simulink model "Quadrocopter_control"  (Simulink 7.4)
settings: Solver=ode45  StartTime=0.0  StopTime=10.0  RelTol=1e-3
values from neighbouring files (symbols this model uses):
  f1 = (I_y-I_z)/I_x    [quadrocopter_param.m]
  f2 = rot.J_z/I_x    [quadrocopter_param.m]
  f3 = (I_z-I_x)/I_y    [quadrocopter_param.m]
  f4 = rot.J_z/I_y    [quadrocopter_param.m]
  f5 = (I_x-I_y)/I_z    [quadrocopter_param.m]
  g = 9.81    [quadrocopter_param.m]
  I_x = elec.I_x+bat.I_x+2*boom.I_1x+2*boom.I_1y+2*mot.I_1x+2*mot.I_1y+                             2*rot.I_1x+2*rot.I_1y    [quadrocopter_param.m]
  I_y = elec.I_y+bat.I_y+2*boom.I_1x+2*boom.I_1y+2*mot.I_1x+2*mot.I_1y+                             2*rot.I_1x+2*rot.I_1y    [quadrocopter_param.m]
  I_z = elec.I_z+bat.I_z+4*boom.I_1z+4*mot.I_1z+4*rot.I_1z    [quadrocopter_param.m]
  m = m*1.2    [quadrocopter_param.m]
  phi0 = 0.15    [Quadrocopter_control_Driver.m]    (also in calc_stability.m = 0; control_two_angles_Driver.m; control_two_angles_and_yawrate_Driver.m; discrete_control_phi_theta_rpsi_Driver.m)
  r_phi0 = 0    [Quadrocopter_control_Driver.m]    (also in calc_stability.m; control_two_angles_Driver.m; control_two_angles_and_yawrate_Driver.m; discrete_control_phi_theta_rpsi_Driver.m)
  r_psi0 = 0    [Quadrocopter_control_Driver.m]    (also in calc_stability.m; control_two_angles_Driver.m = 0.01; control_two_angles_and_yawrate_Driver.m = 0.01; discrete_control_phi_theta_rpsi_Driver.m = 0.01)
  r_theta0 = 0    [Quadrocopter_control_Driver.m]    (also in calc_stability.m; control_two_angles_Driver.m; control_two_angles_and_yawrate_Driver.m; discrete_control_phi_theta_rpsi_Driver.m)
  theta0 = 0.15    [Quadrocopter_control_Driver.m]    (also in calc_stability.m = 0; control_two_angles_Driver.m; control_two_angles_and_yawrate_Driver.m; discrete_control_phi_theta_rpsi_Driver.m)
  Ts = 0.005    [quadrocopter_param.m]
undefined symbols (not defined in the file or in its folder): boom, DiscIntNeverNeededParam
libraries: Copter_Library x4, Control_lib x2, simulink x1
settings Model: Creator=roczit00  LastModifiedBy=roczit00

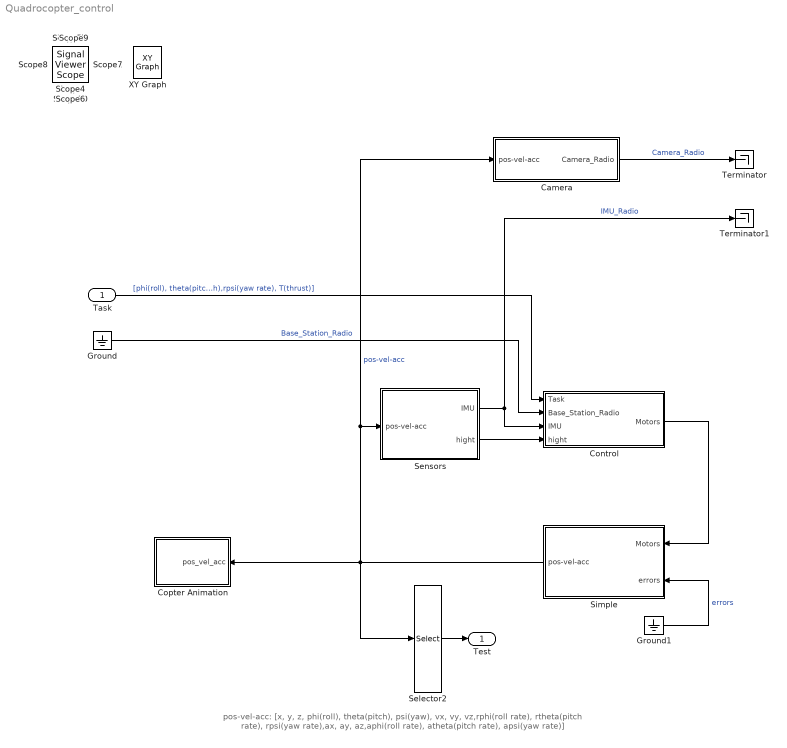
== system Quadrocopter_control ==
  note: pos-vel-acc: [x, y, z, phi(roll), theta(pitch), psi(yaw), vx, vy, vz,rphi(roll rate), rtheta(pitch rate), rpsi(yaw rate),ax, ay, az,aphi(roll rate), atheta(pitch rate), apsi(yaw rate)]
  Task : Inport  PortDimensions=4  OutDataType=fixdt(1, 16)  OutScaling=2^0
  Camera : Subsystem
  Control : Subsystem
  Copter Animation : Subsystem  mask(Quadrocopter Animation){AXES=[-100 100 -100 100 0 100], T_INT=1/25, K_VAR=Feste Position, K_POS=[5 0 1], K_ANGLE=27, A_ON=on, u_phi=on, u_theta=on, u_psi=on, u_x=off, u_y=off, u_z=off}
      mask prompts: AXES "Achsen Grenzen [xmin xmax ymin ymax zmin zmax]"; T_INT "Zeitintervall zwischen Aktualisierungen [s]:"; K_VAR "Kamera Art:"; K_POS "Ort der Kamera [xc yc zc]:"; K_ANGLE "Öffnungswinkel der Kamera [Grad]:"; A_ON "Animation Einschalten:"; u_phi "Use Input phi:"; u_theta "Use Input theta:"; u_psi "Use Input psi:"; u_x "Use Input x:"; u_y "Use Input y:"; u_z "Use Input z:"
      mask help: Erstellt eine 3-D animierte Ansicht eines Quadrocopters.
      mask init:
      | Config.axes = AXES;
      | Config.update = T_INT;
      | Config.camera_view = K_VAR;
      | Config.camera_pos = K_POS;
      | Config.view = K_ANGLE;
      | Config.Animenable = A_ON;
      | Config.phi = u_phi;
      | Config.theta = u_theta;
      | Config.psi = u_psi;
      | Config.x = u_x;
      | Config.y = u_y;
      | Config.z = u_z;
      mask Help:
      | <p>Dieser Block erstellt ein 3 dimensionales Fenster eines Quadrocopters.
      | 
      | <p><H4>Block Eingänge</H4>
      | Der Eingangsvektor bestehend aus:
      | <ul>
      | <li>X-Koordinate - Ort bezogen auf die X-Achse
      | <li>Y-Koordinate - Ort bezogen auf die Y-Achse
      | <li>Z-Koordinate - Ort bezogen auf die Z-Achse
      | <li>Psi - Yaw Drehung um die Z-Achse
      | <li>Phi - Roll Drehen um die Achse in Flugrichtung
      | <li>theta - pitch Neigung in Flugrichtung nach oben bzw. unten
      | </ul></p>
      mask StyleString: edit,edit,popup(Feste Position|Frei bewegbar),edit,edit,checkbox,checkbox,checkbox,checkbox,checkbox,checkbox,checkbox
  Ground : Ground
  Ground1 : Ground
  Selector2 : Selector  InputPortWidth=18  IndexOptions=Index vector (dialog)  Indices=[3 4 5 6]  OutputSizes=1
  Sensors : Subsystem
  Simple : Subsystem  AncestorBlock=Control_lib/Simple
  Terminator : Terminator
  Terminator1 : Terminator
  Test : Outport  OutDataType=fixdt(1, 16)  OutScaling=2^0
  Scope : SignalViewerScope  IOType=viewer  ZoomMode=yonly  LegendLocations="960.3333           681           100      67.33333"  RefreshTime=0.035000
      settings: ShowLegends=on
  Scope1 : SignalViewerScope  IOType=viewer  ZoomMode=yonly  LegendLocations="1037.3333            687             82      67.333333"  RefreshTime=0.035000
      settings: ShowLegends=on
  Scope10 : SignalViewerScope  IOType=viewer  ZoomMode=yonly  LegendLocations="549.3333      405.3333           118            46"  RefreshTime=0.035000
      settings: ShowLegends=on  SaveName=ScopeData10
  Scope2 : SignalViewerScope  IOType=viewer  ZoomMode=yonly  RefreshTime=0.035000
      settings: ShowLegends=on  SaveName=ScopeData2
  Scope3 : SignalViewerScope  IOType=viewer  LegendLocations="235.3333           136            72      67.33333"  RefreshTime=0.035000
      settings: ShowLegends=on  SaveName=ScopeData3
  Scope4 : SignalViewerScope  IOType=viewer  RefreshTime=0.035000
      settings: ShowLegends=on  SaveName=ScopeData4
  Scope5 : SignalViewerScope  IOType=viewer  LegendLocations="401.3333      415.6667           173      192.6667"  RefreshTime=0.035000
      settings: ShowLegends=on  SaveName=ScopeData5
  Scope6 : SignalViewerScope  IOType=viewer  RefreshTime=0.035000
      settings: ShowLegends=on  SaveName=ScopeData6
  Scope7 : SignalViewerScope  IOType=viewer  ZoomMode=yonly  RefreshTime=0.035000
      settings: SaveName=ScopeData7
  Scope8 : SignalViewerScope  IOType=viewer  ZoomMode=yonly  LegendLocations="553.3333      502.3333            92            41"  RefreshTime=0.035000
      settings: ShowLegends=on  SaveName=ScopeData8
  Scope9 : SignalViewerScope  IOType=viewer  LegendLocations="167.3333      162.3333           127            41"  RefreshTime=0.035000
      settings: ShowLegends=on  SaveName=ScopeData9
  XY Graph : simulink/Sinks/XY Graph  IOType=viewer  SystemSampleTime=-1  xmin=-1  xmax=1  ymin=-1  ymax=1  st=-1
  wires:
  Sensors/1(IMU) -> Control/3(IMU), Terminator1/1  "IMU_Radio"
  Sensors/2(hight) -> Control/4(hight)
  Ground1/1 -> Simple/2(errors)  "errors"
  Control/1(Motors) -> Simple/1(Motors)
  Simple/1(pos-vel-acc) -> Sensors/1(pos-vel-acc), Camera/1(pos-vel-acc), Selector2/1, Copter Animation/1(pos_vel_acc)  "pos-vel-acc"
  Camera/1(Camera_Radio) -> Terminator/1  "Camera_Radio"
  Ground/1 -> Control/2(Base_Station_Radio)  "Base_Station_Radio"
  Task/1 -> Control/1(Task)  "[phi(roll), theta(pitch),rpsi(yaw rate), T(thrust)]"
  Selector2/1 -> Test/1

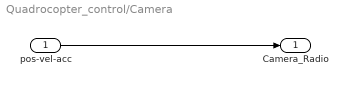
== system Quadrocopter_control/Camera ==
  pos-vel-acc : Inport  OutDataType=fixdt(1, 16)  OutScaling=2^0
  Camera_Radio : Outport  OutDataType=fixdt(1, 16)  OutScaling=2^0
  wires:
  pos-vel-acc/1 -> Camera_Radio/1

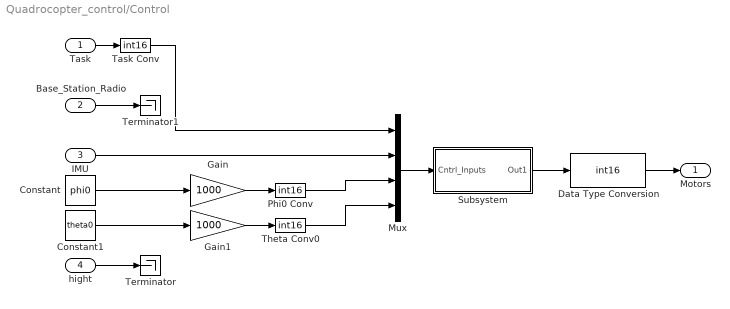
== system Quadrocopter_control/Control ==
  Task : Inport  PortDimensions=4  DataType=double  OutDataType=fixdt(1, 16)  OutScaling=2^0  OutDataTypeStr=double
  Base_Station_Radio : Inport  Port=2  OutDataType=fixdt(1, 16)  OutScaling=2^0
  IMU : Inport  Port=3  DataType=int16  OutDataType=fixdt(1, 16)  OutScaling=2^0  OutDataTypeStr=int16
  hight : Inport  Port=4  DataType=int16  OutDataType=fixdt(1, 16)  OutScaling=2^0  OutDataTypeStr=int16
  Constant : Constant  Value=phi0  OutDataType=fixdt(1, 16)  OutScaling=2^0
  Constant1 : Constant  Value=theta0  OutDataType=fixdt(1, 16)  OutScaling=2^0
  Data Type Conversion : DataTypeConversion  OutDataTypeMode=int16  OutDataType=fixdt(1, 16)  OutScaling=2^0  OutDataTypeStr=int16
  Gain : Gain  Gain=1000  ParameterDataType=fixdt(1, 16)  ParameterScaling=2^0  OutDataType=fixdt(1, 16)  OutScaling=2^0
  Gain1 : Gain  Gain=1000  ParameterDataType=fixdt(1, 16)  ParameterScaling=2^0  OutDataType=fixdt(1, 16)  OutScaling=2^0
  Mux : Mux
  Phi0 Conv : DataTypeConversion  OutDataTypeMode=int16  OutDataType=fixdt(1, 16)  OutScaling=2^0  OutDataTypeStr=int16
  Subsystem : Subsystem  AncestorBlock=Control_lib/Subsystem  mask{G=9.81}
      mask prompts: G "Erdbeschleunigung [m/s²]:"
      mask init:
      | g = G;
  Task Conv : DataTypeConversion  OutDataTypeMode=int16  OutDataType=fixdt(1, 16)  OutScaling=2^0  OutDataTypeStr=int16
  Terminator : Terminator
  Terminator1 : Terminator
  Theta Conv0 : DataTypeConversion  OutDataTypeMode=int16  OutDataType=fixdt(1, 16)  OutScaling=2^0  OutDataTypeStr=int16
  Motors : Outport  PortDimensions=4  DataType=int16  OutDataType=fixdt(1, 16)  OutScaling=2^0  OutDataTypeStr=int16
  wires:
  Base_Station_Radio/1 -> Terminator1/1
  hight/1 -> Terminator/1
  IMU/1 -> Mux/2
  Mux/1 -> Subsystem/1(Cntrl_Inputs)
  Data Type Conversion/1 -> Motors/1
  Subsystem/1(Out1) -> Data Type Conversion/1
  Task/1 -> Task Conv/1
  Task Conv/1 -> Mux/1
  Constant/1 -> Gain/1
  Constant1/1 -> Gain1/1
  Gain/1 -> Phi0 Conv/1
  Gain1/1 -> Theta Conv0/1
  Phi0 Conv/1 -> Mux/3
  Theta Conv0/1 -> Mux/4

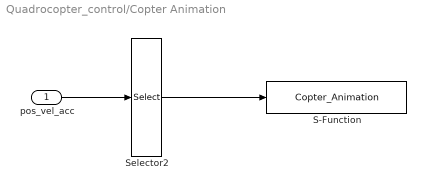
== system Quadrocopter_control/Copter Animation ==
  pos_vel_acc : Inport  PortDimensions=18  OutDataType=sfix(16)  OutScaling=2^0
  S-Function : S-Function  FunctionName=Copter_Animation  Parameters=Config  EnableBusSupport=off
  Selector2 : Selector  InputPortWidth=18  IndexOptions=Index vector (dialog)  Indices=[1 2 3 4 5 6]  OutputSizes=1
  wires:
  pos_vel_acc/1 -> Selector2/1
  Selector2/1 -> S-Function/1

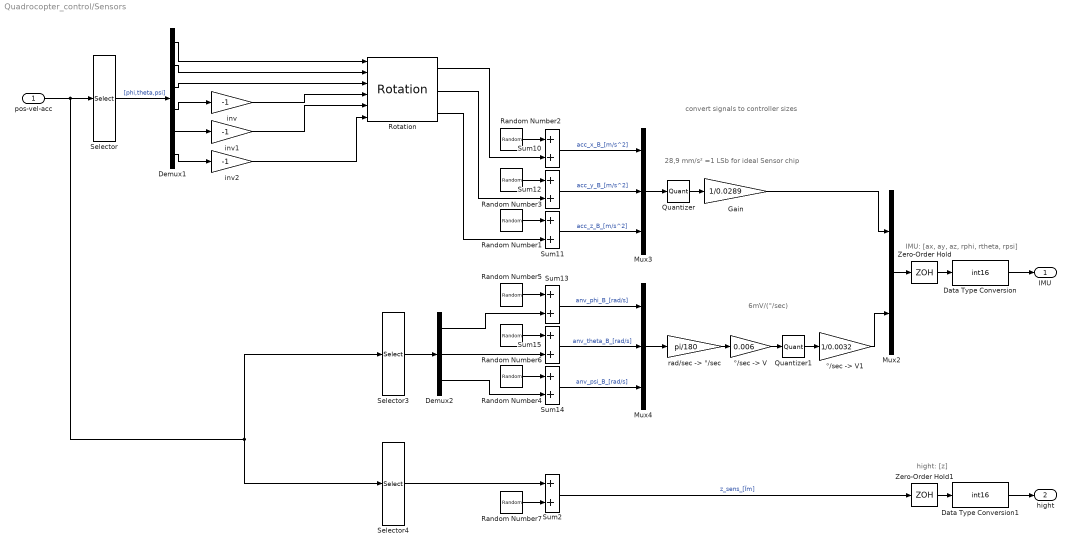
== system Quadrocopter_control/Sensors ==
  note: IMU: [ax, ay, az, rphi, rtheta, rpsi]
  note: hight: [z]
  note: convert signals to controller sizes
  note: 28,9 mm/s² =1 LSb for ideal Sensor chip
  note: 6mV/(°/sec)
  pos-vel-acc : Inport  PortDimensions=18  OutDataType=fixdt(1, 16)  OutScaling=2^0
  Data Type Conversion : DataTypeConversion  OutDataTypeMode=int16  OutDataType=fixdt(1, 16)  OutScaling=2^0  OutDataTypeStr=int16  RndMeth=Round
  Data Type Conversion1 : DataTypeConversion  OutDataTypeMode=int16  OutDataType=fixdt(1, 16)  OutScaling=2^0  OutDataTypeStr=int16  RndMeth=Round
  Demux1 : Demux  Outputs=6
  Demux2 : Demux  Outputs=3
  Gain : Gain  Gain=1/0.0289  ParameterDataType=fixdt(1, 16)  ParameterScaling=2^0  OutDataType=fixdt(1, 16)  OutScaling=2^0
  Mux2 : Mux  Inputs=2
  Mux3 : Mux  Inputs=3
  Mux4 : Mux  Inputs=3
  Quantizer : Quantizer  QuantizationInterval=0.0289
  Quantizer1 : Quantizer  QuantizationInterval=0.0032
  Random Number1 : RandomNumber  Variance=0.0018105  Seed=4684684654  SampleTime=Ts
  Random Number2 : RandomNumber  Variance=0.0003  Seed=456456465  SampleTime=0.01
  Random Number3 : RandomNumber  Variance=0.0003  Seed=676764  SampleTime=Ts
  Random Number{4..7} (4 alike) : RandomNumber  Variance=0  SampleTime=Ts
  Rotation : Control_lib/Rotation  SystemSampleTime=-1
  Selector : Selector  InputPortWidth=18  IndexOptions=Index vector (dialog)  Indices=[13 14 15 4 5 6]  OutputSizes=1
  Selector3 : Selector  InputPortWidth=18  IndexOptions=Index vector (dialog)  Indices=[10 11 12]  OutputSizes=1
  Selector4 : Selector  InputPortWidth=18  IndexOptions=Index vector (dialog)  Indices=[3]  OutputSizes=1
  Sum{2,10..15} (7 alike) : Sum  OutDataType=fixdt(1, 16)  OutScaling=2^0
  Zero-Order Hold : ZeroOrderHold  SampleTime=Ts
  Zero-Order Hold1 : ZeroOrderHold  SampleTime=Ts
  inv : Gain  Gain=-1  ParameterDataType=fixdt(1, 16)  ParameterScaling=2^0  OutDataType=fixdt(1, 16)  OutScaling=2^0
  inv1 : Gain  Gain=-1  ParameterDataType=fixdt(1, 16)  ParameterScaling=2^0  OutDataType=fixdt(1, 16)  OutScaling=2^0
  inv2 : Gain  Gain=-1  ParameterDataType=fixdt(1, 16)  ParameterScaling=2^0  OutDataType=fixdt(1, 16)  OutScaling=2^0
  "rad/sec -> °/sec" : Gain  Gain=pi/180  ParameterDataType=fixdt(1, 16)  ParameterScaling=2^0  OutDataType=fixdt(1, 16)  OutScaling=2^0
  "°/sec -> V" : Gain  Gain=0.006  ParameterDataType=fixdt(1, 16)  ParameterScaling=2^0  OutDataType=fixdt(1, 16)  OutScaling=2^0
  "°/sec -> V1" : Gain  Gain=1/0.0032  ParameterDataType=fixdt(1, 16)  ParameterScaling=2^0  OutDataType=fixdt(1, 16)  OutScaling=2^0
  IMU : Outport  OutDataType=fixdt(1, 16)  OutScaling=2^0
  hight : Outport  Port=2  OutDataType=fixdt(1, 16)  OutScaling=2^0
  wires:
  Random Number7/1 -> Sum2/2
  Random Number2/1 -> Sum10/1
  Random Number1/1 -> Sum11/1
  Random Number3/1 -> Sum12/1
  Random Number5/1 -> Sum13/1
  Random Number4/1 -> Sum14/1
  Random Number6/1 -> Sum15/1
  Demux2/2 -> Sum15/2
  pos-vel-acc/1 -> Selector/1, Selector4/1, Selector3/1
  Selector/1 -> Demux1/1  "[phi,theta,psi]"
  Selector4/1 -> Sum2/1
  Demux2/1 -> Sum13/2
  Demux2/3 -> Sum14/2
  Selector3/1 -> Demux2/1
  Mux2/1 -> Zero-Order Hold/1
  Sum2/1 -> Zero-Order Hold1/1  "z_sens_[Ïm]"
  Zero-Order Hold1/1 -> Data Type Conversion1/1
  Data Type Conversion1/1 -> hight/1
  Zero-Order Hold/1 -> Data Type Conversion/1
  Data Type Conversion/1 -> IMU/1
  Sum10/1 -> Mux3/1  "acc_x_B_[m/s^2]"
  Sum12/1 -> Mux3/2  "acc_y_B_[m/s^2]"
  Sum11/1 -> Mux3/3  "acc_z_B_[m/s^2]"
  Sum13/1 -> Mux4/1  "anv_phi_B_[rad/s]"
  Sum15/1 -> Mux4/2  "anv_theta_B_[rad/s]"
  Sum14/1 -> Mux4/3  "anv_psi_B_[rad/s]"
  Mux3/1 -> Quantizer/1
  Quantizer/1 -> Gain/1
  Gain/1 -> Mux2/1
  "°/sec -> V1"/1 -> Mux2/2
  Mux4/1 -> "rad/sec -> °/sec"/1
  "rad/sec -> °/sec"/1 -> "°/sec -> V"/1
  Quantizer1/1 -> "°/sec -> V1"/1
  "°/sec -> V"/1 -> Quantizer1/1
  Demux1/1 -> Rotation/1
  Demux1/2 -> Rotation/2
  Demux1/3 -> Rotation/3
  Rotation/1 -> Sum10/2
  Rotation/2 -> Sum12/2
  Rotation/3 -> Sum11/2
  Demux1/4 -> inv/1
  Demux1/5 -> inv1/1
  Demux1/6 -> inv2/1
  inv/1 -> Rotation/4
  inv1/1 -> Rotation/5
  inv2/1 -> Rotation/6

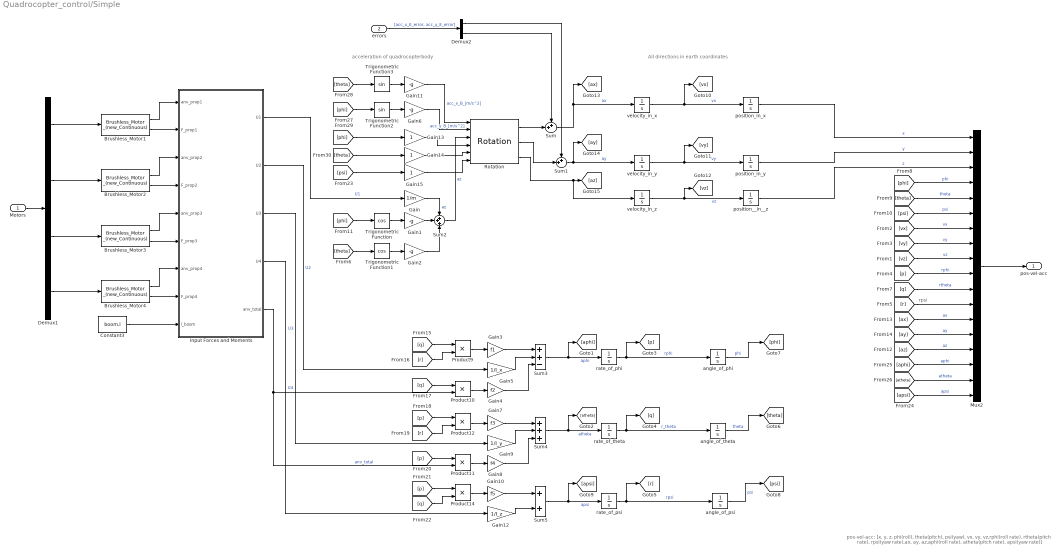
== system Quadrocopter_control/Simple ==
  note: rpsi
  note: pos-vel-acc: [x, y, z, phi(roll), theta(pitch), psi(yaw), vx, vy, vz,rphi(roll rate), rtheta(pitch rate), rpsi(yaw rate),ax, ay, az,aphi(roll rate), atheta(pitch rate), apsi(yaw rate)]
  note: All directions in earth coordinates
  note: acceleration of quadrocopterbody
  Motors : Inport  OutDataType=fixdt(1, 16)  OutScaling=2^0
  errors : Inport  Port=2  OutDataType=fixdt(1, 16)  OutScaling=2^0
  Brushless_Motor{1..4} (4 alike) : Copter_Library/Brushless_Motor _(new_Continuous)  SystemSampleTime=-1  M_error=0
  Constant3 : Constant  Value=boom.l  OutDataType=fixdt(1, 16)  OutScaling=2^0
  Demux1 : Demux
  Demux2 : Demux  Outputs=2
  Gain : Gain  Gain=1/m  ParameterDataType=fixdt(1, 16)  ParameterScaling=2^0  OutDataType=fixdt(1, 16)  OutScaling=2^0
  Gain{1..2,6,11} (4 alike) : Gain  Gain=-g  ParameterDataType=fixdt(1, 16)  ParameterScaling=2^0  OutDataType=fixdt(1, 16)  OutScaling=2^0
  Gain10 : Gain  Gain=f5  ParameterDataType=fixdt(1, 16)  ParameterScaling=2^0  OutDataType=fixdt(1, 16)  OutScaling=2^0
  Gain12 : Gain  Gain=1/I_z  ParameterDataType=fixdt(1, 16)  ParameterScaling=2^0  OutDataType=fixdt(1, 16)  OutScaling=2^0
  Gain13 : Gain  ParameterDataType=fixdt(1, 16)  ParameterScaling=2^0  OutDataType=fixdt(1, 16)  OutScaling=2^0
  Gain14 : Gain  ParameterDataType=fixdt(1, 16)  ParameterScaling=2^0  OutDataType=fixdt(1, 16)  OutScaling=2^0
  Gain15 : Gain  ParameterDataType=fixdt(1, 16)  ParameterScaling=2^0  OutDataType=fixdt(1, 16)  OutScaling=2^0
  Gain3 : Gain  Gain=f1  ParameterDataType=fixdt(1, 16)  ParameterScaling=2^0  OutDataType=fixdt(1, 16)  OutScaling=2^0
  Gain4 : Gain  Gain=f2  ParameterDataType=fixdt(1, 16)  ParameterScaling=2^0  OutDataType=fixdt(1, 16)  OutScaling=2^0
  Gain5 : Gain  Gain=1/I_x  ParameterDataType=fixdt(1, 16)  ParameterScaling=2^0  OutDataType=fixdt(1, 16)  OutScaling=2^0
  Gain7 : Gain  Gain=f3  ParameterDataType=fixdt(1, 16)  ParameterScaling=2^0  OutDataType=fixdt(1, 16)  OutScaling=2^0
  Gain8 : Gain  Gain=f4  ParameterDataType=fixdt(1, 16)  ParameterScaling=2^0  OutDataType=fixdt(1, 16)  OutScaling=2^0
  Gain9 : Gain  Gain=1/I_y  ParameterDataType=fixdt(1, 16)  ParameterScaling=2^0  OutDataType=fixdt(1, 16)  OutScaling=2^0
  Input Forces and Moments : Stateflow chart
  Mux2 : Mux  Inputs=18
  Product{9..12,14} (5 alike) : Product  OutDataType=fixdt(1, 16)  OutScaling=2^0  RndMeth=Zero
  Rotation : Control_lib/Rotation  SystemSampleTime=-1
  Sum : Sum  Inputs=++|  OutDataType=fixdt(1, 16)  OutScaling=2^0
  Sum1 : Sum  Inputs=++|  OutDataType=fixdt(1, 16)  OutScaling=2^0
  Sum2 : Sum  Inputs=+++  OutDataType=fixdt(1, 16)  OutScaling=2^0
  Sum3 : Sum  Inputs=++-  OutDataType=fixdt(1, 16)  OutScaling=2^0
  Sum4 : Sum  Inputs=+++  OutDataType=fixdt(1, 16)  OutScaling=2^0
  Sum5 : Sum  OutDataType=fixdt(1, 16)  OutScaling=2^0
  Trigonometric Function : Trigonometry  Operator=cos
  Trigonometric Function1 : Trigonometry  Operator=cos
  Trigonometric Function2 : Trigonometry
  Trigonometric Function3 : Trigonometry
  angle_of_phi : Integrator  InitialCondition=phi0
  angle_of_psi : Integrator
  angle_of_theta : Integrator  InitialCondition=theta0
  position__in__z : Integrator
  position_in_x : Integrator
  position_in_y : Integrator
  rate_of_phi : Integrator  InitialCondition=r_phi0
  rate_of_psi : Integrator  InitialCondition=r_psi0
  rate_of_theta : Integrator  InitialCondition=r_theta0
  velocity_in_x : Integrator
  velocity_in_y : Integrator
  velocity_in_z : Integrator
  pos-vel-acc : Outport  OutDataType=fixdt(1, 16)  OutScaling=2^0
  wires:
  [apsi] -> Mux2/18  "apsi"
  [atheta] -> Mux2/17  "atheta"
  [aphi] -> Mux2/16  "aphi"
  [az] -> Mux2/15  "az"
  [ay] -> Mux2/14  "ay"
  [ax] -> Mux2/13  "ax"
  [r] -> Mux2/12
  [q] -> Mux2/11  "rtheta"
  [p] -> Mux2/10  "rphi"
  [vz] -> Mux2/9  "vz"
  [vy] -> Mux2/8  "vy"
  [vx] -> Mux2/7  "vx"
  [psi] -> Mux2/6  "psi"
  [theta] -> Mux2/5  "theta"
  [phi] -> Mux2/4  "phi"
  position__in__z/1 -> Mux2/3  "z"
  Mux2/1 -> pos-vel-acc/1
  errors/1 -> Demux2/1  "[acc_x_E_error, acc_y_E_error]"
  Motors/1 -> Demux1/1
  Demux1/3 -> Brushless_Motor3/1
  Demux1/4 -> Brushless_Motor4/1
  Demux1/2 -> Brushless_Motor2/1
  Demux1/1 -> Brushless_Motor1/1
  velocity_in_x/1 -> [vx], position_in_x/1  "vx"
  velocity_in_y/1 -> [vy], position_in_y/1  "vy"
  velocity_in_z/1 -> [vz], position__in__z/1  "vz"
  Constant3/1 -> Input Forces and Moments/9(l_boom)
  Sum5/1 -> [apsi], rate_of_psi/1  "apsi"
  Input Forces and Moments/4(U4) -> Gain12/1  "U4"
  Gain12/1 -> Sum5/2
  Gain10/1 -> Sum5/1
  Product14/1 -> Gain10/1
  [q] -> Product14/2
  [p] -> Product14/1
  Sum4/1 -> [atheta], rate_of_theta/1  "atheta"
  Input Forces and Moments/3(U3) -> Gain9/1  "U3"
  Gain8/1 -> Sum4/3
  Gain9/1 -> Sum4/2
  Product11/1 -> Gain8/1
  [p] -> Product11/1
  Gain7/1 -> Sum4/1
  Product12/1 -> Gain7/1
  [r] -> Product12/2
  [p] -> Product12/1
  Input Forces and Moments/1(U1) -> Gain/1  "U1"
  Sum3/1 -> [aphi], rate_of_phi/1  "aphi"
  Gain4/1 -> Sum3/3
  Gain5/1 -> Sum3/2
  Input Forces and Moments/2(U2) -> Gain5/1  "U2"
  Product10/1 -> Gain4/1
  [q] -> Product10/1
  Gain3/1 -> Sum3/1
  Product9/1 -> Gain3/1
  [r] -> Product9/2
  [q] -> Product9/1
  Input Forces and Moments/5(anv_total) -> Product11/2, Product10/2  "anv_total"
  angle_of_phi/1 -> [phi]  "phi"
  angle_of_theta/1 -> [theta]  "theta"
  angle_of_psi/1 -> [psi]  "psi"
  rate_of_phi/1 -> [p], angle_of_phi/1  "rphi"
  rate_of_theta/1 -> angle_of_theta/1, [q]  "r_theta"
  rate_of_psi/1 -> angle_of_psi/1, [r]  "rpsi"
  Brushless_Motor1/1 -> Input Forces and Moments/1(anv_prop1)
  Brushless_Motor1/2 -> Input Forces and Moments/2(F_prop1)
  Brushless_Motor2/1 -> Input Forces and Moments/3(anv_prop2)
  Brushless_Motor2/2 -> Input Forces and Moments/4(F_prop2)
  Brushless_Motor3/1 -> Input Forces and Moments/5(anv_prop3)
  Brushless_Motor3/2 -> Input Forces and Moments/6(F_prop3)
  Brushless_Motor4/1 -> Input Forces and Moments/7(anv_prop4)
  Brushless_Motor4/2 -> Input Forces and Moments/8(F_prop4)
  position_in_x/1 -> Mux2/1  "x"
  position_in_y/1 -> Mux2/2  "y"
  Sum1/1 -> [ay], velocity_in_y/1  "ay"
  Sum/1 -> [ax], velocity_in_x/1  "ax"
  Demux2/2 -> Sum/1
  Demux2/1 -> Sum1/1
  Gain/1 -> Sum2/1  "az"
  Gain1/1 -> Sum2/2
  Gain2/1 -> Sum2/3
  [phi] -> Trigonometric Function/1
  [theta] -> Trigonometric Function1/1
  Trigonometric Function/1 -> Gain1/1
  Trigonometric Function1/1 -> Gain2/1
  [phi] -> Trigonometric Function2/1
  Trigonometric Function2/1 -> Gain6/1
  [theta] -> Trigonometric Function3/1
  Trigonometric Function3/1 -> Gain11/1
  Rotation/3 -> [az], velocity_in_z/1
  Rotation/2 -> Sum1/2
  Rotation/1 -> Sum/2
  Gain11/1 -> Rotation/1  "acc_x_B_[m/s^2]"
  Gain6/1 -> Rotation/2  "acc_y_B_[m/s^2]"
  Sum2/1 -> Rotation/3  "az"
  [phi] -> Gain13/1
  [theta] -> Gain14/1
  [psi] -> Gain15/1
  Gain13/1 -> Rotation/4
  Gain14/1 -> Rotation/5
  Gain15/1 -> Rotation/6

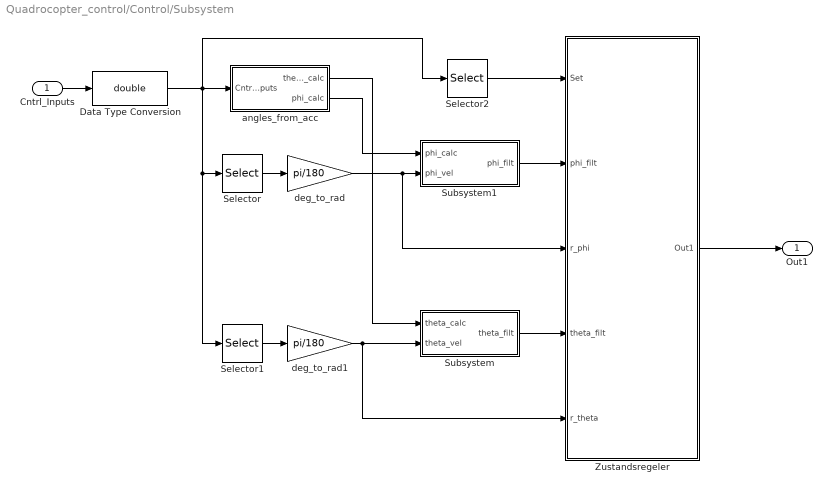
== system Quadrocopter_control/Control/Subsystem ==
  Cntrl_Inputs : Inport  OutDataType=fixdt(1, 16)  OutScaling=2^0
  Data Type Conversion : DataTypeConversion  OutDataTypeMode=double  OutDataType=fixdt(1, 16)  OutScaling=2^0  OutDataTypeStr=double
  Selector : Selector  InputPortWidth=12  IndexOptions=Index vector (dialog)  Indices=[8]  OutputSizes=1
  Selector1 : Selector  InputPortWidth=12  IndexOptions=Index vector (dialog)  Indices=[9]  OutputSizes=1
  Selector2 : Selector  InputPortWidth=12  IndexOptions=Index vector (dialog)  Indices=[1 2 3 4]  OutputSizes=1
  Subsystem : Subsystem
  Subsystem1 : Subsystem
  Zustandsregeler : Subsystem  mask{FB_phi=-10, FB_r_phi=-10, FB_theta=-10, FB_r_theta=-10}
      mask prompts: FB_phi "Feedbackfactor phi:"; FB_r_phi "Feedbackfactor r_phi:"; FB_theta "Feedbackfactor theta:"; FB_r_theta "Feedbackfactor theta:"
  angles_from_acc : Subsystem  mask{g=g}
      mask prompts: g "Erdbeschleunigung [m/s²]:"
  deg_to_rad : Gain  Gain=pi/180  ParameterDataType=fixdt(1, 16)  ParameterScaling=2^0  OutDataType=fixdt(1, 16)  OutScaling=2^0  SampleTime=10
  deg_to_rad1 : Gain  Gain=pi/180  ParameterDataType=fixdt(1, 16)  ParameterScaling=2^0  OutDataType=fixdt(1, 16)  OutScaling=2^0  SampleTime=10
  Out1 : Outport  OutDataType=fixdt(1, 16)  OutScaling=2^0
  wires:
  Subsystem/1(theta_filt) -> Zustandsregeler/4(theta_filt)
  Subsystem1/1(phi_filt) -> Zustandsregeler/2(phi_filt)
  Zustandsregeler/1(Out1) -> Out1/1
  deg_to_rad1/1 -> Zustandsregeler/5(r_theta), Subsystem/2(theta_vel)
  Selector1/1 -> deg_to_rad1/1
  deg_to_rad/1 -> Zustandsregeler/3(r_phi), Subsystem1/2(phi_vel)
  Selector/1 -> deg_to_rad/1
  Data Type Conversion/1 -> Selector1/1, Selector/1, Selector2/1, angles_from_acc/1(Cntrl_Inputs)
  Cntrl_Inputs/1 -> Data Type Conversion/1
  Selector2/1 -> Zustandsregeler/1(Set)
  angles_from_acc/1(theta_calc) -> Subsystem/1(theta_calc)
  angles_from_acc/2(phi_calc) -> Subsystem1/1(phi_calc)

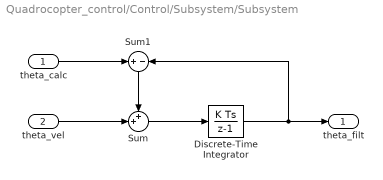
== system Quadrocopter_control/Control/Subsystem/Subsystem ==
  theta_calc : Inport  OutDataType=fixdt(1, 16)  OutScaling=2^0
  theta_vel : Inport  Port=2  OutDataType=fixdt(1, 16)  OutScaling=2^0
  Discrete-Time Integrator : DiscreteIntegrator  InitialCondition=theta0  SampleTime=Ts  OutDataType=fixdt(1, 16)  OutScaling=2^0  ICPrevOutput=DiscIntNeverNeededParam  ICPrevScaledInput=DiscIntNeverNeededParam
  Sum : Sum  Inputs=++|  OutDataType=fixdt(1, 16)  OutScaling=2^0
  Sum1 : Sum  Inputs=+|-  OutDataType=fixdt(1, 16)  OutScaling=2^0
  theta_filt : Outport  OutDataType=fixdt(1, 16)  OutScaling=2^0
  wires:
  theta_calc/1 -> Sum1/1
  Sum1/1 -> Sum/1
  theta_vel/1 -> Sum/2
  Sum/1 -> Discrete-Time Integrator/1
  Discrete-Time Integrator/1 -> Sum1/2, theta_filt/1

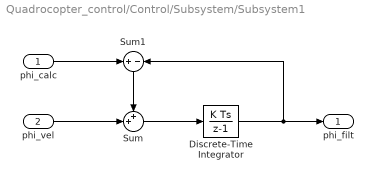
== system Quadrocopter_control/Control/Subsystem/Subsystem1 ==
  phi_calc : Inport  OutDataType=fixdt(1, 16)  OutScaling=2^0
  phi_vel : Inport  Port=2  OutDataType=fixdt(1, 16)  OutScaling=2^0
  Discrete-Time Integrator : DiscreteIntegrator  InitialCondition=theta0  SampleTime=Ts  OutDataType=fixdt(1, 16)  OutScaling=2^0  ICPrevOutput=DiscIntNeverNeededParam  ICPrevScaledInput=DiscIntNeverNeededParam
  Sum : Sum  Inputs=++|  OutDataType=fixdt(1, 16)  OutScaling=2^0
  Sum1 : Sum  Inputs=+|-  OutDataType=fixdt(1, 16)  OutScaling=2^0
  phi_filt : Outport  OutDataType=fixdt(1, 16)  OutScaling=2^0
  wires:
  phi_calc/1 -> Sum1/1
  Sum1/1 -> Sum/1
  phi_vel/1 -> Sum/2
  Sum/1 -> Discrete-Time Integrator/1
  Discrete-Time Integrator/1 -> Sum1/2, phi_filt/1

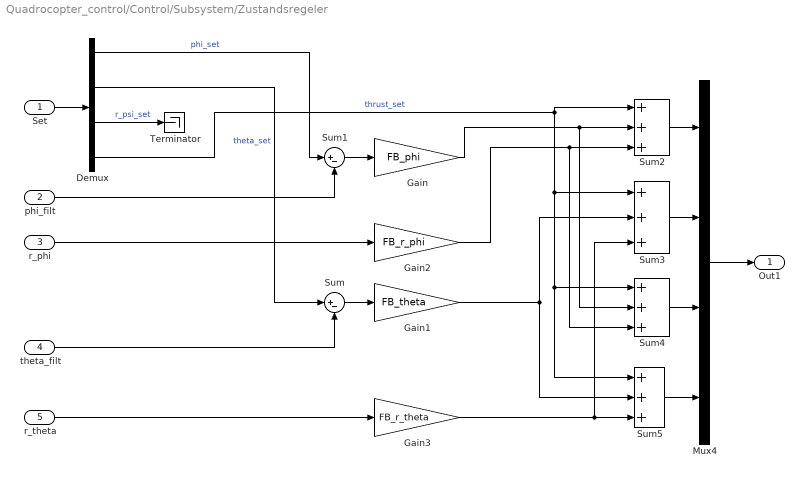
== system Quadrocopter_control/Control/Subsystem/Zustandsregeler ==
  Set : Inport  OutDataType=fixdt(1, 16)  OutScaling=2^0
  phi_filt : Inport  Port=2  OutDataType=fixdt(1, 16)  OutScaling=2^0
  r_phi : Inport  Port=3  OutDataType=fixdt(1, 16)  OutScaling=2^0
  theta_filt : Inport  Port=4  OutDataType=fixdt(1, 16)  OutScaling=2^0
  r_theta : Inport  Port=5  OutDataType=fixdt(1, 16)  OutScaling=2^0
  Demux : Demux
  Gain : Gain  Gain=FB_phi  ParameterDataType=fixdt(1, 16)  ParameterScaling=2^0  OutDataType=fixdt(1, 16)  OutScaling=2^0
  Gain1 : Gain  Gain=FB_theta  ParameterDataType=fixdt(1, 16)  ParameterScaling=2^0  OutDataType=fixdt(1, 16)  OutScaling=2^0
  Gain2 : Gain  Gain=FB_r_phi  ParameterDataType=fixdt(1, 16)  ParameterScaling=2^0  OutDataType=fixdt(1, 16)  OutScaling=2^0
  Gain3 : Gain  Gain=FB_r_theta  ParameterDataType=fixdt(1, 16)  ParameterScaling=2^0  OutDataType=fixdt(1, 16)  OutScaling=2^0
  Mux4 : Mux
  Sum : Sum  Inputs=|+-  OutDataType=fixdt(1, 16)  OutScaling=2^0
  Sum1 : Sum  Inputs=|+-  OutDataType=fixdt(1, 16)  OutScaling=2^0
  Sum{2..5} (4 alike) : Sum  Inputs=+++  OutDataType=fixdt(1, 16)  OutScaling=2^0
  Terminator : Terminator
  Out1 : Outport  OutDataType=fixdt(1, 16)  OutScaling=2^0
  wires:
  Demux/4 -> Sum3/1, Sum5/1, Sum4/1, Sum2/1  "thrust_set"
  Demux/3 -> Terminator/1  "r_psi_set"
  r_theta/1 -> Gain3/1
  theta_filt/1 -> Sum/2
  r_phi/1 -> Gain2/1
  phi_filt/1 -> Sum1/2
  Demux/2 -> Sum/1  "theta_set"
  Demux/1 -> Sum1/1  "phi_set"
  Set/1 -> Demux/1
  Gain3/1 -> Sum3/3, Sum5/3
  Gain2/1 -> Sum4/3, Sum2/3
  Sum/1 -> Gain1/1
  Gain1/1 -> Sum3/2, Sum5/2
  Gain/1 -> Sum4/2, Sum2/2
  Sum1/1 -> Gain/1
  Sum5/1 -> Mux4/4
  Sum4/1 -> Mux4/3
  Sum3/1 -> Mux4/2
  Sum2/1 -> Mux4/1
  Mux4/1 -> Out1/1

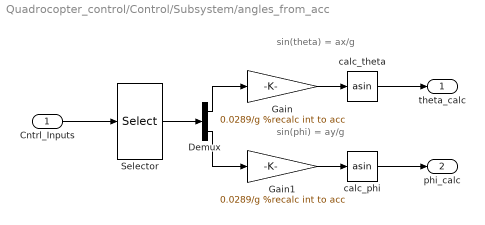
== system Quadrocopter_control/Control/Subsystem/angles_from_acc ==
  note: sin(theta) = ax/g
  note: sin(phi) = ay/g
  Cntrl_Inputs : Inport  OutDataType=fixdt(1, 16)  OutScaling=2^0
  Demux : Demux  Outputs=2
  Gain : Gain  Gain=0.0289/g %recalc int to acc  ParameterDataType=fixdt(1, 16)  ParameterScaling=2^0  OutDataType=fixdt(1, 16)  OutScaling=2^0
  Gain1 : Gain  Gain=0.0289/g %recalc int to acc  ParameterDataType=fixdt(1, 16)  ParameterScaling=2^0  OutDataType=fixdt(1, 16)  OutScaling=2^0
  Selector : Selector  InputPortWidth=12  IndexOptions=Index vector (dialog)  Indices=[5 6 ]  OutputSizes=1
  calc_phi : Trigonometry  Operator=asin
  calc_theta : Trigonometry  Operator=asin
  theta_calc : Outport  OutDataType=fixdt(1, 16)  OutScaling=2^0
  phi_calc : Outport  Port=2  OutDataType=fixdt(1, 16)  OutScaling=2^0
  wires:
  Gain1/1 -> calc_phi/1
  Demux/2 -> Gain1/1
  Gain/1 -> calc_theta/1
  Demux/1 -> Gain/1
  calc_phi/1 -> phi_calc/1
  calc_theta/1 -> theta_calc/1
  Selector/1 -> Demux/1
  Cntrl_Inputs/1 -> Selector/1

== matlab function Simple/Input Forces and Moments ==
  data: anv_prop1 input double; F_prop1 input double; anv_prop2 input double; F_prop2 input double; anv_prop3 input double; F_prop3 input double; anv_prop4 input double; U1 output double; F_prop4 input double; U2 output double; U3 output double; U4 output double; l_boom input double; anv_total output double
function [U1, U2, U3, U4, anv_total] = input(anv_prop1,F_prop1,anv_prop2,...
    F_prop2,anv_prop3,F_prop3,anv_prop4,F_prop4,l_boom)
%#eml

% Calculating Thrust in z-axis with respect to body fixed coordinate system
U1 = F_prop1 + F_prop2 + F_prop3 + F_prop4;             % [N]

% Calculating Torque around x-axis (Roll) due to Thrust
U2 = l_boom*(-F_prop4+F_prop2);                         % [Nm]

% Calculating Torque around y-axis (Pitch) due to Thrust
U3 = l_boom*(-F_prop1+F_prop3);                         % [Nm]

% Calculating Torque around z-axis (Yaw) due to Thrust
U4 = l_boom*(F_prop1-F_prop2+F_prop3-F_prop4);          % [Nm]

% Overall propeller speed
anv_total = anv_prop1-anv_prop2+anv_prop3-anv_prop4;    % [rad/s]
